simulink model "lab4_"  (R2021b)
settings: Solver=ode4  StartTime=0.0  StopTime=10.0  FixedStep=2^-7  RelTol=1e-3
libraries: simulink x1
settings Model: Creator=JaSzw  LastModifiedBy=JaSzw

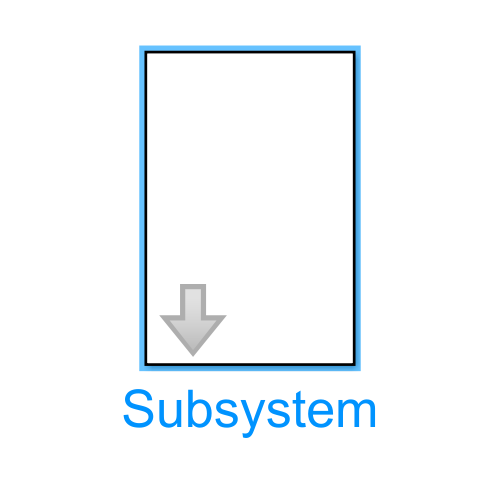
[thumbnail: Simulink's stored preview of the top-level diagram]
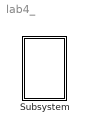
== system lab4_ ==
  Subsystem : Subsystem  mask{M=200, R=2, rs=0.2, G=9.81, x0=0, xv=10, y0=5, yv=0}
      mask prompts: M "masa planety"; R "promien planety"; rs "promien satelity"; G "przyspieszenie grawitacyjne"

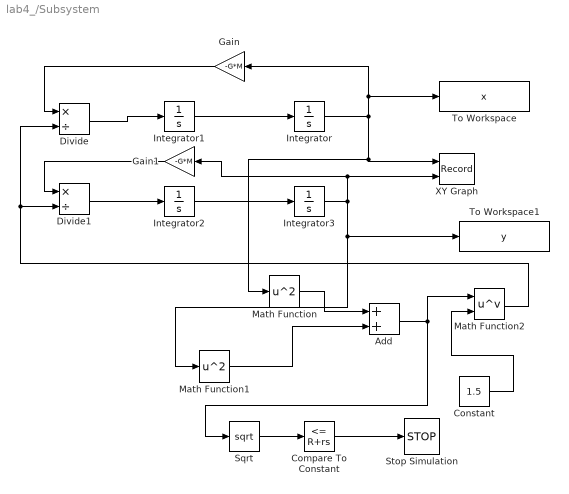
== system lab4_/Subsystem ==
  Add : Sum
  Compare To Constant : simulink/Logic and Bit Operations/Compare To Constant  relop=<=  const=R+rs  OutDataTypeStr=boolean
  Constant : Constant  Value=1.5
  Divide : Product  Inputs=*/
  Divide1 : Product  Inputs=*/
  Gain : Gain  Gain=-G*M
  Gain1 : Gain  Gain=-G*M
  Integrator : Integrator  InitialCondition=x0
  Integrator1 : Integrator  InitialCondition=xv
  Integrator2 : Integrator  InitialCondition=yv
  Integrator3 : Integrator  InitialCondition=y0
  Math Function : Math  Operator=square  SaturateOnIntegerOverflow=on
  Math Function1 : Math  Operator=square  SaturateOnIntegerOverflow=on
  Math Function2 : Math  Operator=pow  SaturateOnIntegerOverflow=on
  Sqrt : Sqrt  SaturateOnIntegerOverflow=on
  Stop Simulation : Stop
  To Workspace : ToWorkspace  VariableName=x  SampleTime=-1
  To Workspace1 : ToWorkspace  VariableName=y  SampleTime=-1
  XY Graph : Record  FileSettingsInternal="{\"entries\":[{\"content\":{\"excelSettings\":{\"content\":{},\"type\":\"Streamout.ExcelSettings\"}},\"type\":\"Streamout.FileSettingStorage\",\"uuid\":\"e5b2dbb4-b533-48e5-b3bd-0913e113d32f\"}],\"packageUris\":[\"http://schema.mathworks.com/mf0/streamout_blocks/R2020a\"],\"version\":\"1.0\"}"  Layout=[1 1]  SignalsInternal="{\"entries\":[{\"content\":{\"signals\":[{\"content\":{\"blockPath\":[\"lab4_/Subsystem/XY Graph\"],\"channel\":[],\"dimensions\":[1],\"domain\":\"lab4_/Subsystem/XY Graph\",\"lineColor\":\"#a2142f\",\"plots\":[1],\"port\":1,\"sid\":[\"\"],\"signalID\":141,\"signalName\":\"Integrator\"},\"type\":\"RecordBlkView.Signal\",\"uuid\":\"c9e3d9ff-d5b6-40d1-95bf-fe7348a11828\"},{\"content\":{\"blockPath\":[\"lab4_/Subsystem/XY Graph\"],\"channel\":[],\"dimensions\":[1],\"domain\":\"lab4_/Subsystem/XY Graph\",\"lineColor\":\"#139fff\",\"plots\":[1],\"port\":2,\"sid\":[\"\"],\"signalID\":145,\"signalName\":\"Integrator3\"},\"type\":\"RecordBlkView.Signal\",\"uuid\":\"ef67189c-1484-461f-a674-78f72259a665\"}]},\"type\":\"RecordBlkView.InputSignals\",\"uuid\":\"97ac483b-663c-4598-befc-e07817f1f420\"}],\"packageUris\":[\"http://schema.mathworks.com/mf0/streamout_blocks/R2020a\"],\"version\":\"1.0\"}"  VisualizationBindings="{\"xyplotplugin\":{\"info\":[{\"series\":[{\"bindingParametersList\":[{\"parameter\":\"X-Axis\",\"signalID\":141,\"signalName\":\"Integrator\"},{\"parameter\":\"Y-Axis\",\"signalID\":145,\"signalName\":\"Integrator3\"}],\"seriesID\":39551}],\"subplotID\":1}]}}"  CompatibilityTag=XY
  wires:
  Integrator3/1 -> XY Graph/2, Gain1/1, Math Function1/1, To Workspace1/1
  Math Function/1 -> Add/1
  Integrator1/1 -> Integrator/1
  Sqrt/1 -> Compare To Constant/1
  Integrator2/1 -> Integrator3/1
  Integrator/1 -> XY Graph/1, Math Function/1, To Workspace/1, Gain/1
  Constant/1 -> Math Function2/2
  Math Function2/1 -> Divide1/2, Divide/2
  Gain1/1 -> Divide1/1
  Gain/1 -> Divide/1
  Compare To Constant/1 -> Stop Simulation/1
  Divide1/1 -> Integrator2/1
  Divide/1 -> Integrator1/1
  Math Function1/1 -> Add/2
  Add/1 -> Sqrt/1, Math Function2/1
